simulink model "hw1"  (R2019a)
settings: Solver=VariableStepAuto  StartTime=0.0  StopTime=10.0  RelTol=1e-3
settings Model: Creator=sumli  LastModifiedBy=sumli

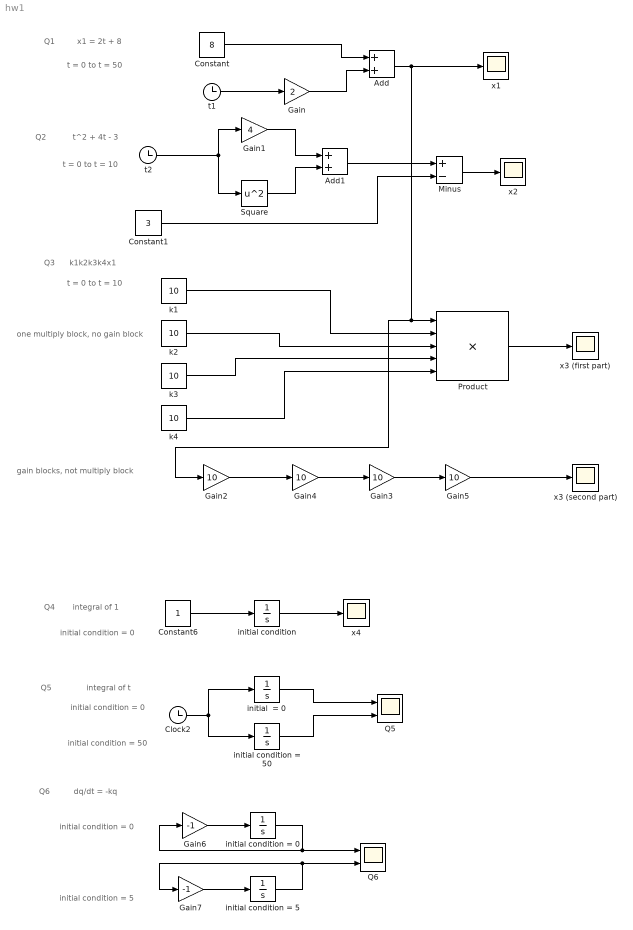
== system hw1 ==
  note: gain blocks, not multiply block
  note: initial condition = 5
  note: initial condition = 0
  note: dq/dt = -kq
  note: Q6
  note: initial condition = 50
  note: initial condition = 0
  note: integral of t
  note: Q5
  note: initial condition = 0
  note: integral of 1
  note: Q4
  note: one multiply block, no gain block
  note: t = 0 to t = 10
  note: k1k2k3k4x1
  note: Q3
  note: t = 0 to t = 10
  note: t = 0 to t = 50
  note: t^2 + 4t - 3
  note: x1 = 2t + 8
  note: Q2
  note: Q1
  Add : Sum
  Add1 : Sum
  Clock2 : Clock
  Constant : Constant  Value=8
  Constant1 : Constant  Value=3
  Constant6 : Constant
  Gain : Gain  Gain=2
  Gain1 : Gain  Gain=4
  Gain{2..5} (4 alike) : Gain  Gain=10
  Gain6 : Gain  Gain=-1
  Gain7 : Gain  Gain=-1
  Minus : Sum  Inputs=+-
  Product : Product  Inputs=5
  "Q5 " : Scope  NumInputPorts=2
  Q6 : Scope  NumInputPorts=2
  Square : Math  Operator=square  SaturateOnIntegerOverflow=on
  "initial  = 0 " : Integrator
  initial condition : Integrator
  initial condition = 0 : Integrator
  initial condition = 5 : Integrator  InitialCondition=5
  initial condition = 50 : Integrator  InitialCondition=50
  k{1..4} (4 alike) : Constant  Value=10
  t1 : Clock
  t2 : Clock
  x1 : Scope
  "x2 " : Scope
  x3 (first part) : Scope
  x3 (second part) : Scope
  "x4 " : Scope
  wires:
  t1/1 -> Gain/1
  Constant/1 -> Add/1
  Gain/1 -> Add/2
  Add/1 -> Gain2/1, Product/1, x1/1
  t2/1 -> Square/1, Gain1/1
  Gain1/1 -> Add1/1
  Square/1 -> Add1/2
  Add1/1 -> Minus/1
  Constant1/1 -> Minus/2
  Minus/1 -> "x2 "/1
  k4/1 -> Product/5
  k3/1 -> Product/4
  k2/1 -> Product/3
  k1/1 -> Product/2
  Product/1 -> x3 (first part)/1
  Gain2/1 -> Gain4/1
  Gain4/1 -> Gain3/1
  Gain3/1 -> Gain5/1
  Gain5/1 -> x3 (second part)/1
  Constant6/1 -> initial condition/1
  initial condition/1 -> "x4 "/1
  Clock2/1 -> "initial  = 0 "/1, initial condition = 50/1
  initial condition = 50/1 -> "Q5 "/2
  "initial  = 0 "/1 -> "Q5 "/1
  initial condition = 0/1 -> Gain6/1, Q6/1
  initial condition = 5/1 -> Gain7/1, Q6/2
  Gain6/1 -> initial condition = 0/1
  Gain7/1 -> initial condition = 5/1
